simulink model "Power_Subsystem_Designer"  (R2022b)
settings: Solver=VariableStepAuto  StartTime=0.0  StopTime=1  MaxStep=0.0001  RelTol=1e-3
undefined symbols (not defined in the file): ABS_MAX_TORQUE, ABS_MIN_TORQUE, dTx, MAX_MOTOR_CURRENT, min_velocity_regen, MOTOR_ENABLE, motorControllerCurve, motorTempCurve, motorTempX, throttleCurve, throttleX
libraries: simulink x1
settings Model: Creator=Inver  LastModifiedBy=dagge
settings ModelReferenceCC: EnableRefExpFcnMdlSchedulingChecks=on

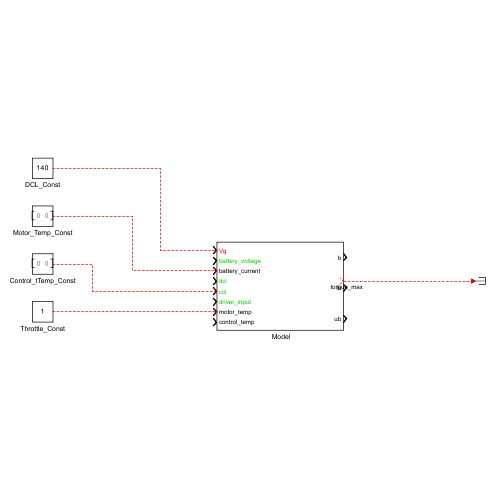
[thumbnail: Simulink's stored preview of the top-level diagram]
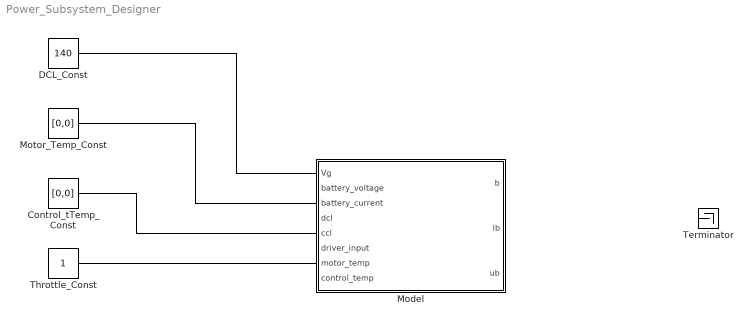
== system Power_Subsystem_Designer ==
  " Model" : Subsystem
  Control_tTemp_Const : Constant  Value=[0,0]
  DCL_Const : Constant  Value=140  SampleTime=10
  Motor_Temp_Const : Constant  Value=[0,0]
  Terminator : Terminator
  Throttle_Const : Constant
  wires:
  ? -> Terminator/1  "torque_max"
  DCL_Const/1 -> ?
  Control_tTemp_Const/1 -> ?
  Motor_Temp_Const/1 -> ?
  Throttle_Const/1 -> ?

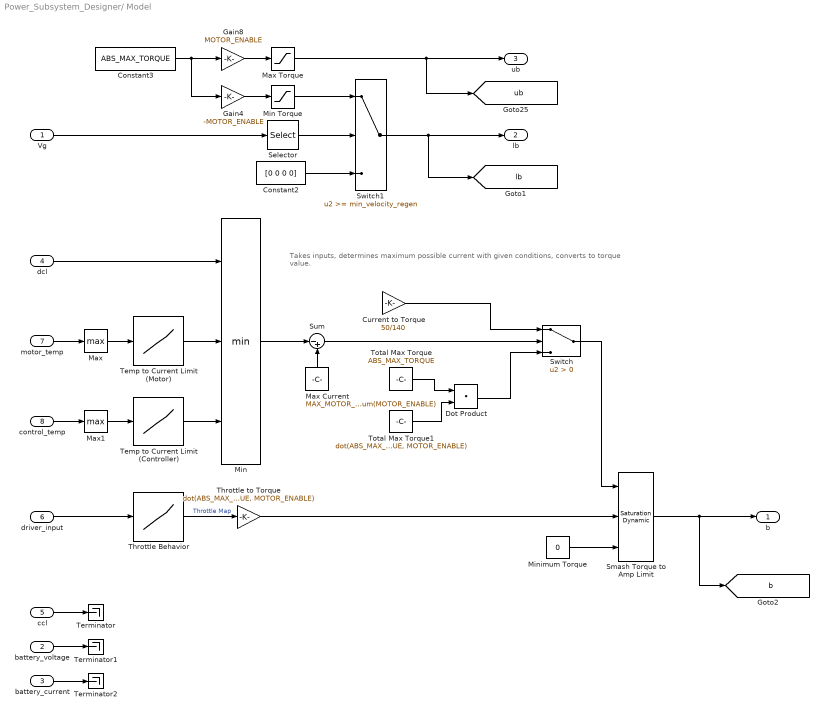
== system Power_Subsystem_Designer/ Model ==
  note: Takes inputs, determines maximum possible current with given conditions, converts to torque value.
  Vg : Inport  OutDataTypeStr=double
  battery_voltage : Inport  Port=2
  battery_current : Inport  Port=3
  dcl : Inport  Port=4  OutDataTypeStr=double  LockScale=on
  ccl : Inport  Port=5  OutDataTypeStr=double  LockScale=on
  driver_input : Inport  Port=6  OutDataTypeStr=double  LockScale=on
  motor_temp : Inport  Port=7
  control_temp : Inport  Port=8
  Constant2 : Constant  Value=[0 0 0 0]  OutDataTypeStr=double
  Constant3 : Constant  Value=ABS_MAX_TORQUE
  Current to Torque : Gain  Gain=50/140
  Dot Product : DotProduct  OutDataTypeStr=Inherit: Inherit via internal rule
  Gain4 : Gain  Gain=-MOTOR_ENABLE  ParamDataTypeStr=double  OutDataTypeStr=Inherit: Inherit via back propagation
  Gain8 : Gain  Gain=MOTOR_ENABLE  ParamDataTypeStr=double  OutDataTypeStr=Inherit: Inherit via back propagation
  Max : MinMax  Function=max
  Max Current : Constant  Value=MAX_MOTOR_CURRENT * sum(MOTOR_ENABLE)
  Max Torque : Saturate  UpperLimit=ABS_MAX_TORQUE  LowerLimit=dTx  OutDataTypeStr=Inherit: Inherit via back propagation
  Max1 : MinMax  Function=max
  Min : MinMax  Inputs=3
  Min Torque : Saturate  UpperLimit=0  LowerLimit=ABS_MIN_TORQUE  OutDataTypeStr=Inherit: Inherit via back propagation
  "Minimum Torque " : Constant  Value=0
  Selector : Selector  InputPortWidth=4  IndexOptions=Index vector (dialog)  Indices=4  OutputSizes=1
  Smash Torque to Amp Limit : simulink/Discontinuities/Saturation Dynamic  OutMin=[0]  OutMax=[]  OutDataTypeStr=Inherit: Same as second input  OutDataType=fixdt(1, 16)  OutScaling=2^-10  DoSatur=off
  Sum : Sum  Inputs=|-+
  Switch : Switch  Criteria=u2 > Threshold  SaturateOnIntegerOverflow=off  InputSameDT=off
  Switch1 : Switch  Threshold=min_velocity_regen  OutDataTypeStr=Inherit: Inherit via back propagation  SaturateOnIntegerOverflow=off  InputSameDT=off
  Temp to Current Limit (Controller) : Lookup_n-D  NumberOfTableDimensions=1  BreakpointsForDimension1=motorControllerCurve(:,1)  IndexSearchMethod=Evenly spaced points  Table=motorControllerCurve(:,2)  ExtrapMethod=Clip  UseLastTableValue=on  InternalRulePriority=Speed  RndMeth=Simplest
  Temp to Current Limit (Motor) : Lookup_n-D  NumberOfTableDimensions=1  BreakpointsForDimension1=motorTempX  IndexSearchMethod=Evenly spaced points  Table=motorTempCurve  ExtrapMethod=Clip  UseLastTableValue=on  InternalRulePriority=Speed  RndMeth=Simplest
  Terminator : Terminator
  Terminator1 : Terminator
  Terminator2 : Terminator
  "Throttle Behavior " : Lookup_n-D  NumberOfTableDimensions=1  BreakpointsForDimension1=throttleX  IndexSearchMethod=Evenly spaced points  Table=throttleCurve  InternalRulePriority=Speed  RndMeth=Simplest
  Throttle to Torque : Gain  Gain=dot(ABS_MAX_TORQUE, MOTOR_ENABLE)
  Total Max Torque : Constant  Value=ABS_MAX_TORQUE
  Total Max Torque1 : Constant  Value=dot(ABS_MAX_TORQUE, MOTOR_ENABLE)
  b : Outport  OutDataTypeStr=double  LockScale=on
  lb : Outport  Port=2  OutDataTypeStr=double  LockScale=on
  ub : Outport  Port=3  OutDataTypeStr=double  LockScale=on
  tag scope: b=global, lb=global, ub=global
  wires:
  Sum/1 -> Switch/2
  Switch/1 -> Smash Torque to Amp Limit/1
  Min/1 -> Sum/1
  Dot Product/1 -> Switch/3
  Total Max Torque1/1 -> Dot Product/2
  Current to Torque/1 -> Switch/1
  Constant3/1 -> Gain4/1, Gain8/1
  "Minimum Torque "/1 -> Smash Torque to Amp Limit/3
  Min Torque/1 -> Switch1/1
  driver_input/1 -> "Throttle Behavior "/1
  Switch1/1 -> [lb], lb/1
  battery_voltage/1 -> Terminator1/1
  "Throttle Behavior "/1 -> Throttle to Torque/1  "Throttle Map"
  control_temp/1 -> Max1/1
  Max Current/1 -> Sum/2
  Smash Torque to Amp Limit/1 -> b/1, [b]
  Throttle to Torque/1 -> Smash Torque to Amp Limit/2
  Max Torque/1 -> [ub], ub/1
  Max1/1 -> Temp to Current Limit (Controller)/1
  Total Max Torque/1 -> Dot Product/1
  battery_current/1 -> Terminator2/1
  Constant2/1 -> Switch1/3
  dcl/1 -> Min/1
  Gain8/1 -> Max Torque/1
  Vg/1 -> Selector/1
  Selector/1 -> Switch1/2
  Temp to Current Limit (Motor)/1 -> Min/2
  Temp to Current Limit (Controller)/1 -> Min/3
  ccl/1 -> Terminator/1
  Gain4/1 -> Min Torque/1
  Max/1 -> Temp to Current Limit (Motor)/1
  motor_temp/1 -> Max/1
